simulink model "Project_sb"  (R2021a)
settings: Solver=VariableStepAuto  StartTime=0.0  StopTime=10
InitFcn:
  | t_switch = 2;
  | t_switch_rev = 5;
  | t_trans = 1;
  | c_st_fr = 0.3;
  | c_dyn_fr = 0.3;
  | kp_w = 100;
  | ki_w = 100;
  | kd_w = 100;
model workspace: external: MATLAB File C:\Users\SPb19\Desktop\project\export\Project_sb_DataFile.m (data not in the file)
undefined symbols (not defined in the file or in its folder): h, smiData, w, X, Y, Z
libraries: sm_lib x173, nesl_utility x23, pid_lib x7
(part 6 of 6)

== system Project_sb/Wheel_2/link2_t3_1_w2 ==
  ReferenceFrame : sm_lib/Frames and Transforms/Reference Frame
  Solid : sm_lib/Body Elements/File Solid  ExtGeomFileName=link2.stp_Default_sldprt.STEP  UnitType=FromFile  ExtGeomFileUnits=m  StepReaderType=HEX  ExportConvexHullGeometry=off  InertiaType=Custom  Mass=smiData.Solid(1).mass  MassUnits=kg  CenterOfMass=smiData.Solid(1).CoM  CenterOfMassUnits=mm  MomentsOfInertia=smiData.Solid(1).MoI  MomentsOfInertiaUnits=kg*mm^2  ProductsOfInertia=smiData.Solid(1).PoI  ProductsOfInertiaUnits=kg*mm^2  BasedOnType=DensityFromFile  Density=1000  DensityUnits=kg/m^3  DoExposeReferenceFrame=on  SerializedFrames=<Frames/>  GraphicType=FromGeometry  MarkerShape=Sphere  MarkerSize=10  GraphicVisPropType=SimpleVisualProperties  GraphicDiffuseColor=[0.0 0.4 1.0]  GraphicSpecularColor=[0.5 0.5 0.5 1.0]  GraphicAmbientColor=[0.15 0.15 0.15 1.0]  GraphicEmissiveColor=[0.0 0.0 0.0 1.0]  GraphicShininess=75  GraphicOpacity=smiData.Solid(1).opacity
  Transform : sm_lib/Frames and Transforms/Rigid Transform  TranslationMethod=Cartesian  TranslationStandardOffset=0  TranslationLengthUnit=mm  TranslationStandardAxis=+Z  TranslationCartesianOffset=smiData.RigidTransform(1).translation  TranslationROffset=0  TranslationROffsetUnits=m  TranslationZOffset=0  TranslationZOffsetUnits=m  TranslationThetaOffset=0  TranslationThetaOffsetUnits=deg  RotationMethod=ArbitraryAxis  RotationAngleUnits=rad  RotationStandardAxis=+Z  RotationAngle=smiData.RigidTransform(1).angle  RotationArbitraryAxis=smiData.RigidTransform(1).axis  FollAlignAxisA=+X  BaseAlignAxisA=+Y  FollAlignAxisB=+Y  BaseAlignAxisB=+Z  RotationSequenceAxes=FollowerAxes  RotationSequence=XYX  RotationSequenceAngles=[0 0 0]  RotationSequenceAnglesUnits=deg  RotationMatrix=[1 0 0; 0 1 0; 0 0 1]
  Transform1 : sm_lib/Frames and Transforms/Rigid Transform  TranslationMethod=Cartesian  TranslationStandardOffset=0  TranslationLengthUnit=mm  TranslationStandardAxis=+Z  TranslationCartesianOffset=smiData.RigidTransform(14).translation  TranslationROffset=0  TranslationROffsetUnits=m  TranslationZOffset=0  TranslationZOffsetUnits=m  TranslationThetaOffset=0  TranslationThetaOffsetUnits=deg  RotationMethod=ArbitraryAxis  RotationAngleUnits=rad  RotationStandardAxis=+Z  RotationAngle=smiData.RigidTransform(14).angle  RotationArbitraryAxis=smiData.RigidTransform(14).axis  FollAlignAxisA=+X  BaseAlignAxisA=+Y  FollAlignAxisB=+Y  BaseAlignAxisB=+Z  RotationSequenceAxes=FollowerAxes  RotationSequence=XYX  RotationSequenceAngles=[0 0 0]  RotationSequenceAnglesUnits=deg  RotationMatrix=[1 0 0; 0 1 0; 0 0 1]
  F1 : PMIOPort  Side=Left
  F : PMIOPort  Port=2  Side=Right
  connections:
  Solid/RConn1 -- ReferenceFrame/RConn1 -- Transform/LConn1 -- Transform1/LConn1
  Transform/RConn1 -- F/RConn1
  Transform1/RConn1 -- F1/RConn1

== system Project_sb/Wheel_2/link2_t3_2_w2 ==
  ReferenceFrame : sm_lib/Frames and Transforms/Reference Frame
  Solid : sm_lib/Body Elements/File Solid  ExtGeomFileName=link2.stp_Default_sldprt.STEP  UnitType=FromFile  ExtGeomFileUnits=m  StepReaderType=HEX  ExportConvexHullGeometry=off  InertiaType=Custom  Mass=smiData.Solid(1).mass  MassUnits=kg  CenterOfMass=smiData.Solid(1).CoM  CenterOfMassUnits=mm  MomentsOfInertia=smiData.Solid(1).MoI  MomentsOfInertiaUnits=kg*mm^2  ProductsOfInertia=smiData.Solid(1).PoI  ProductsOfInertiaUnits=kg*mm^2  BasedOnType=DensityFromFile  Density=1000  DensityUnits=kg/m^3  DoExposeReferenceFrame=on  SerializedFrames=<Frames/>  GraphicType=FromGeometry  MarkerShape=Sphere  MarkerSize=10  GraphicVisPropType=SimpleVisualProperties  GraphicDiffuseColor=smiData.Solid(1).color  GraphicSpecularColor=[0.5 0.5 0.5 1.0]  GraphicAmbientColor=[0.15 0.15 0.15 1.0]  GraphicEmissiveColor=[0.0 0.0 0.0 1.0]  GraphicShininess=75  GraphicOpacity=smiData.Solid(1).opacity
  Transform : sm_lib/Frames and Transforms/Rigid Transform  TranslationMethod=Cartesian  TranslationStandardOffset=0  TranslationLengthUnit=mm  TranslationStandardAxis=+Z  TranslationCartesianOffset=smiData.RigidTransform(3).translation  TranslationROffset=0  TranslationROffsetUnits=m  TranslationZOffset=0  TranslationZOffsetUnits=m  TranslationThetaOffset=0  TranslationThetaOffsetUnits=deg  RotationMethod=ArbitraryAxis  RotationAngleUnits=rad  RotationStandardAxis=+Z  RotationAngle=smiData.RigidTransform(3).angle  RotationArbitraryAxis=smiData.RigidTransform(3).axis  FollAlignAxisA=+X  BaseAlignAxisA=+Y  FollAlignAxisB=+Y  BaseAlignAxisB=+Z  RotationSequenceAxes=FollowerAxes  RotationSequence=XYX  RotationSequenceAngles=[0 0 0]  RotationSequenceAnglesUnits=deg  RotationMatrix=[1 0 0; 0 1 0; 0 0 1]
  Transform1 : sm_lib/Frames and Transforms/Rigid Transform  TranslationMethod=Cartesian  TranslationStandardOffset=0  TranslationLengthUnit=mm  TranslationStandardAxis=+Z  TranslationCartesianOffset=smiData.RigidTransform(16).translation  TranslationROffset=0  TranslationROffsetUnits=m  TranslationZOffset=0  TranslationZOffsetUnits=m  TranslationThetaOffset=0  TranslationThetaOffsetUnits=deg  RotationMethod=ArbitraryAxis  RotationAngleUnits=rad  RotationStandardAxis=+Z  RotationAngle=smiData.RigidTransform(16).angle  RotationArbitraryAxis=smiData.RigidTransform(16).axis  FollAlignAxisA=+X  BaseAlignAxisA=+Y  FollAlignAxisB=+Y  BaseAlignAxisB=+Z  RotationSequenceAxes=FollowerAxes  RotationSequence=XYX  RotationSequenceAngles=[0 0 0]  RotationSequenceAnglesUnits=deg  RotationMatrix=[1 0 0; 0 1 0; 0 0 1]
  F1 : PMIOPort  Side=Left
  F : PMIOPort  Port=2  Side=Right
  connections:
  Solid/RConn1 -- ReferenceFrame/RConn1 -- Transform/LConn1 -- Transform1/LConn1
  Transform/RConn1 -- F/RConn1
  Transform1/RConn1 -- F1/RConn1

== matlab function Project_sb/Wheel_1/Subsystem2/MATLAB Function ==
  data: t input; c output; t_switch input; t_switch_rev input; t_trans input
function c = fcn(t,t_switch,t_switch_rev,t_trans)
c0 = -0.665; c1 = -0.9163;
t_lin = linspace(t_switch,t_switch+t_trans,1000);
i = interp1([t_switch,t_switch+t_trans],[c0,c1],t_lin);
t_lin_rev = linspace(t_switch_rev,t_switch_rev+t_trans,1000);
i_rev = interp1([t_switch_rev,t_switch_rev+t_trans],[c1,c0],t_lin_rev);

if t < t_switch
    c = c0;
elseif t_switch <= t && t <= t_switch +t_trans
    c_shh = i(find(abs(t_lin-t) < 1e-1));
    c = c_shh(1);
elseif t_switch +t_trans < t  && t < t_switch_rev
    c = c1;
elseif t_switch_rev <= t && t <= t_switch_rev +t_trans
    c_shh = i_rev(find(abs(t_lin_rev-t) < 1e-1));
    c = c_shh(1);
else
    c = c0;
    
    
    
end

== matlab function Project_sb/Wheel_1/Subsystem/MATLAB Function ==
  data: t input; c output; t_switch input; t_switch_rev input; t_trans input
function c = fcn(t,t_switch,t_switch_rev,t_trans)
c0 = 1.43; c1 = 1.18;
t_lin = linspace(t_switch,t_switch+t_trans,1000);
i = interp1([t_switch,t_switch+t_trans],[c0,c1],t_lin);
t_lin_rev = linspace(t_switch_rev,t_switch_rev+t_trans,1000);
i_rev = interp1([t_switch_rev,t_switch_rev+t_trans],[c1,c0],t_lin_rev);

if t < t_switch
    c = c0;
elseif t_switch <= t && t <= t_switch +t_trans
    c_shh = i(find(abs(t_lin-t) < 1e-1));
    c = c_shh(1);
elseif t_switch +t_trans < t  && t < t_switch_rev
    c = c1;
elseif t_switch_rev <= t && t <= t_switch_rev +t_trans
    c_shh = i_rev(find(abs(t_lin_rev-t) < 1e-1));
    c = c_shh(1);
else
    c = c0;
    
    
    
end

== matlab function Project_sb/Wheel_1/Subsystem1/MATLAB Function ==
  data: t input; c output; t_switch input; t_switch_rev input; t_trans input
function c = fcn(t,t_switch,t_switch_rev,t_trans)
c0 = -2.76; c1 = -3.0107;
t_lin = linspace(t_switch,t_switch+t_trans,1000);
i = interp1([t_switch,t_switch+t_trans],[c0,c1],t_lin);
t_lin_rev = linspace(t_switch_rev,t_switch_rev+t_trans,1000);
i_rev = interp1([t_switch_rev,t_switch_rev+t_trans],[c1,c0],t_lin_rev);

if t < t_switch
    c = c0;
elseif t_switch <= t && t <= t_switch +t_trans
    c_shh = i(find(abs(t_lin-t) < 1e-1));
    c = c_shh(1);
elseif t_switch +t_trans < t  && t < t_switch_rev
    c = c1;
elseif t_switch_rev <= t && t <= t_switch_rev +t_trans
    c_shh = i_rev(find(abs(t_lin_rev-t) < 1e-1));
    c = c_shh(1);
else
    c = c0;
    
    
    
end

== matlab function Project_sb/Wheel_2/Subsystem3/MATLAB Function ==
  data: t input; c output; t_switch input; t_switch_rev input; t_trans input
function c = fcn(t,t_switch,t_switch_rev,t_trans)
c0 = 1.43; c1 = 1.18;
t_lin = linspace(t_switch,t_switch+t_trans,1000);
i = interp1([t_switch,t_switch+t_trans],[c0,c1],t_lin);
t_lin_rev = linspace(t_switch_rev,t_switch_rev+t_trans,1000);
i_rev = interp1([t_switch_rev,t_switch_rev+t_trans],[c1,c0],t_lin_rev);

if t < t_switch
    c = c0;
elseif t_switch <= t && t <= t_switch +t_trans
    c_shh = i(find(abs(t_lin-t) < 1e-1));
    c = c_shh(1);
elseif t_switch +t_trans < t  && t < t_switch_rev
    c = c1;
elseif t_switch_rev <= t && t <= t_switch_rev +t_trans
    c_shh = i_rev(find(abs(t_lin_rev-t) < 1e-1));
    c = c_shh(1);
else
    c = c0;
    
    
    
end

== matlab function Project_sb/Wheel_2/Subsystem5/MATLAB Function ==
  data: t input; c output; t_switch input; t_switch_rev input; t_trans input
function c = fcn(t,t_switch,t_switch_rev,t_trans)
c0 = -0.665; c1 = -0.9163;
t_lin = linspace(t_switch,t_switch+t_trans,1000);
i = interp1([t_switch,t_switch+t_trans],[c0,c1],t_lin);
t_lin_rev = linspace(t_switch_rev,t_switch_rev+t_trans,1000);
i_rev = interp1([t_switch_rev,t_switch_rev+t_trans],[c1,c0],t_lin_rev);

if t < t_switch
    c = c0;
elseif t_switch <= t && t <= t_switch +t_trans
    c_shh = i(find(abs(t_lin-t) < 1e-1));
    c = c_shh(1);
elseif t_switch +t_trans < t  && t < t_switch_rev
    c = c1;
elseif t_switch_rev <= t && t <= t_switch_rev +t_trans
    c_shh = i_rev(find(abs(t_lin_rev-t) < 1e-1));
    c = c_shh(1);
else
    c = c0;
    
    
    
end

== matlab function Project_sb/Wheel_2/Subsystem4/MATLAB Function ==
  data: t input; c output; t_switch input; t_switch_rev input; t_trans input
function c = fcn(t,t_switch,t_switch_rev,t_trans)
c0 = -2.76; c1 = -3.0107;
t_lin = linspace(t_switch,t_switch+t_trans,1000);
i = interp1([t_switch,t_switch+t_trans],[c0,c1],t_lin);
t_lin_rev = linspace(t_switch_rev,t_switch_rev+t_trans,1000);
i_rev = interp1([t_switch_rev,t_switch_rev+t_trans],[c1,c0],t_lin_rev);

if t < t_switch
    c = c0;
elseif t_switch <= t && t <= t_switch +t_trans
    c_shh = i(find(abs(t_lin-t) < 1e-1));
    c = c_shh(1);
elseif t_switch +t_trans < t  && t < t_switch_rev
    c = c1;
elseif t_switch_rev <= t && t <= t_switch_rev +t_trans
    c_shh = i_rev(find(abs(t_lin_rev-t) < 1e-1));
    c = c_shh(1);
else
    c = c0;
    
    
    
end
